simulink model "Modele_LQR_3DOF"  (R2019b)
settings: Solver=VariableStepAuto  StartTime=0.0  StopTime=20  FixedStep=0.1  RelTol=1e-3
undefined symbols (not defined in the file): Amatrix, B, Bmatrix, Fx1, Fx2, Fx3, Fx4, Fx5, Fx6, Fx7, Fx8, Fy1, Fy2, Fy3, Fy4, Fy5, Fy6, Fy7, Fy8, Fz1, Fz2, Fz3, Fz4, Fz5, Fz6, Fz7, Fz8, I_x, I_y, I_z, lx1, lx2, lx3, lx4, lx5, lx6, lx7, lx8, ly1, ly2, ly3, ly4, ly5, ly6, ly7, ly8, lz1, lz2, lz3, lz4, lz5, lz6, lz7, lz8, m, Q, R, W, X0, x_rb ... (+5)
libraries: simulink x12, robotlib x7, dspinverses x1
(part 2 of 2)

== matlab function Modele_LQR_3DOF/ROV model/ROV model/Kinetics1 ==
  data: u input size=1; u_dot output; v input size=1; w input size=1; p input size=1; q input size=1; r input size=1; phi input; theta input; psi input; tau input; v_dot output; w_dot output; p_dot output; q_dot output; r_dot output; u_dot_temp input; v_dot_temp input; w_dot_temp input; p_dot_temp input; q_dot_temp input; r_dot_temp input; disturbance input; EstimatedParams input; B parameter; Fx1 input; Fx2 input; Fx3 input; Fx4 input; Fx5 input; Fx6 input; Fx7 input; Fx8 input; Fy1 input; Fy2 input; Fy3 input; Fy4 input; Fy5 input; Fy6 input; Fy7 input; Fy8 input; Fz1 input; Fz2 input; Fz3 input; Fz4 input; Fz5 input; Fz6 input; Fz7 input; Fz8 input; I_x input; I_y input; I_z input; lx1 input; lx2 input; lx3 input; lx4 input; lx5 input; lx6 input; lx7 input; lx8 input; ly1 input; ly2 input; ly3 input; ly4 input; ly5 input; ly6 input; ly7 input; ly8 input; lz1 input; lz2 input; lz3 input; lz4 input; lz5 input; lz6 input; lz7 input; lz8 input; m parameter; W parameter; x_rb parameter; x_rg parameter; y_rb parameter; y_rg parameter; z_rb parameter; z_rg parameter
function [u_dot,v_dot,w_dot,p_dot,q_dot,r_dot] = Kinetics1(u,v,w,p,q,r,phi,theta,psi,tau,u_dot_temp,v_dot_temp,w_dot_temp,p_dot_temp,q_dot_temp,r_dot_temp, disturbance,EstimatedParams, B, Fx1, Fx2, Fx3, Fx4, Fx5, Fx6, Fx7, Fx8, Fy1, Fy2, Fy3, Fy4, Fy5, Fy6, Fy7, Fy8, Fz1, Fz2, Fz3, Fz4, Fz5, Fz6, Fz7, Fz8, I_x, I_y, I_z, lx1, lx2, lx3, lx4, lx5, lx6, lx7, lx8, ly1, ly2, ly3, ly4, ly5, ly6, ly7, ly8, lz1, lz2, lz3, lz4, lz5, lz6, lz7, lz8, m, W, x_rb, x_rg, y_rb, y_rg, z_rb, z_rg)
% LIVRE HMCH PAGE 58
%extract forces from thrusters
f1=tau(1);
f2=tau(2);
f3=tau(3);
f4=tau(4);
f5=tau(5);
f6=tau(6);
f7=tau(7);
f8=tau(8);

% displaced_water_volume = 0.03;
% water_density = 1000.0;
% m = 24;
% W = -9.81*m;
% B = -W;
%extract estimated parameters
X_u = EstimatedParams(1);
Y_v = EstimatedParams(2);
Z_w = EstimatedParams(3);
K_p = EstimatedParams(4); 
M_q = EstimatedParams(5);
N_r = EstimatedParams(6);
X_uu = EstimatedParams(7);
Y_vv = EstimatedParams(8);
Z_ww = EstimatedParams(9);
K_pp = EstimatedParams(10); 
M_qq = EstimatedParams(11); 
N_rr = EstimatedParams(12);
X_u_dot = EstimatedParams(13);
Y_v_dot = EstimatedParams(14);
Z_w_dot = EstimatedParams(15);
K_p_dot = EstimatedParams(16);
M_q_dot = EstimatedParams(17); 
N_r_dot = EstimatedParams(18); 
%extract forces from disturbance
u_c = disturbance(1);
v_c = disturbance(2);
w_c = disturbance(3);
p_c = disturbance(4);
q_c = disturbance(5);
r_c = disturbance(6);
%Full Equations without disturbance with zg = 0.02
% u_dot = -((0.7071*f1) + (0.7071*f2) - (0.7071*f3) - (0.7071*f4)- (0.230*q_dot_temp) + 2*sin(theta) + u*(X_u + X_uu*abs(u)) - (0.230*p*r) - (11.50*q*w) + (11.50*r*v) - Y_v_dot*r*v + Z_w_dot*q*w)/(X_u_dot - 11.50);
% v_dot = ((0.7071*f1) - (0.7071*f2) + (0.7071*f3) - (0.7071*f4) - (0.230*p_dot_temp) + 2*cos(theta)*sin(phi) - v*(Y_v + Y_vv*abs(v)) + (11.50*q*r) - (11.50*p*w) + (11.50*r*u) - X_u_dot*r*u + Z_w_dot*p*w)/(Y_v_dot - 11.50);
% w_dot = -(f6 - f5 + f7 - f8 - 2*cos(phi)*cos(theta) + w*(Z_w + Z_ww*abs(w)) + q*((23*q)/100 - X_u_dot*u) + p*((23*p)/100 + Y_v_dot*v) - (11.50*p*v) + (11.50*q*u))/(Z_w_dot - 11.50);
% p_dot = -(25*((0.0601*f1) - (0.0601*f2) + (0.0601*f3) - (0.0601*f4) - (109*f5)/500 - (109*f6)/500 + (0.2180*f7) + (0.2180*f8) + (0.230*v_dot_temp) + K_p*p - (2.2560*cos(theta)*sin(phi)) - (0.230*p*w) + (0.230*r*u) - M_q_dot*q*r + N_r_dot*q*r - Y_v_dot*v*w + Z_w_dot*v*w + K_pp*p*abs(p)))/(25*K_p_dot - 4);
% q_dot =-(25*((0.0601*f1) + (0.0601*f2) - (0.0601*f3) - (0.0601*f4)+ (0.120*f5) - (0.120*f6) + (0.120*f7) - (0.120*f8) - (0.230*u_dot_temp) - (2.2560*sin(theta)) + M_q*q - (0.230*q*w) + (0.230*r*v) + K_p_dot*p*r - N_r_dot*p*r + X_u_dot*u*w - Z_w_dot*u*w + M_qq*q*abs(q)))/(25*M_q_dot - 4);
% r_dot = -(25*((0.1888*f2) - (0.1888*f1) + (0.1888*f3) - (0.1888*f4) + N_r*r - K_p_dot*p*q + M_q_dot*p*q - X_u_dot*u*v + Y_v_dot*u*v + N_rr*r*abs(r)))/(25*N_r_dot - 4);

%Full Equations without disturbance with zg = 0.02 + utilisation de la fontion vpa
% u_dot = -(1.0*(0.7071*f1 + 0.7071*f2 - 0.7071*f3 - 0.7071*f4 - 0.23*q_dot_temp + 2.0*sin(theta) + (X_u + X_uu*abs(u - 1.0*u_c))*(u - 1.0*u_c) - 1.0*(11.5*q - 11.5*q_c)*(w - 1.0*w_c) + (11.5*r - 11.5*r_c)*(v - 1.0*v_c) - 1.0*(p - 1.0*p_c)*(0.23*r - 0.23*r_c) + (X_u_dot - 11.5)*(q*w_c - 1.0*r*v_c) - 1.0*Y_v_dot*(r - 1.0*r_c)*(v - 1.0*v_c) + Z_w_dot*(q - 1.0*q_c)*(w - 1.0*w_c)))/(X_u_dot - 11.5);
% v_dot = (0.7071*f1 - 0.7071*f2 + 0.7071*f3 - 0.7071*f4 - 0.23*p_dot_temp - 1.0*(11.5*p - 11.5*p_c)*(w - 1.0*w_c) + (11.5*r - 11.5*r_c)*(u - 1.0*u_c) - 1.0*(Y_v + Y_vv*abs(v - 1.0*v_c))*(v - 1.0*v_c) + 2.0*cos(theta)*sin(phi) + (q - 1.0*q_c)*(0.23*r - 0.23*r_c) + (Y_v_dot - 11.5)*(p*w_c - 1.0*r*u_c) - 1.0*X_u_dot*(r - 1.0*r_c)*(u - 1.0*u_c) + Z_w_dot*(p - 1.0*p_c)*(w - 1.0*w_c))/(Y_v_dot - 11.5);
% w_dot =-(1.0*(f6 - 1.0*f5 + f7 - 1.0*f8 - 1.0*(11.5*p - 11.5*p_c)*(v - 1.0*v_c) + (11.5*q - 11.5*q_c)*(u - 1.0*u_c) - 2.0*cos(phi)*cos(theta) + (Z_w + Z_ww*abs(w - 1.0*w_c))*(w - 1.0*w_c) + (Z_w_dot - 11.5)*(p*v_c - 1.0*q*u_c) + (p - 1.0*p_c)*(0.23*p - 0.23*p_c + Y_v_dot*(v - 1.0*v_c)) - 1.0*(q - 1.0*q_c)*(0.23*q_c - 0.23*q + X_u_dot*(u - 1.0*u_c))))/(Z_w_dot - 11.5);
% p_dot =-(1.0*(0.0601035*f1 - 0.0601035*f2 + 0.0601035*f3 - 0.0601035*f4 - 0.218*f5 - 0.218*f6 + 0.218*f7 + 0.218*f8 + 0.23*v_dot - 2.256*cos(theta)*sin(phi) + (u - 1.0*u_c)*(0.23*r - 0.23*r_c) - 0.23*p*w_c + 0.23*r*u_c - 1.0*(r - 1.0*r_c)*(0.16*q_c - 0.16*q + M_q_dot*(q - 1.0*q_c)) + (q - 1.0*q_c)*(0.16*r_c - 0.16*r + N_r_dot*(r - 1.0*r_c)) + (K_p + K_pp*abs(p - 1.0*p_c))*(p - 1.0*p_c) - 1.0*(w - 1.0*w_c)*(0.23*p - 0.23*p_c + Y_v_dot*(v - 1.0*v_c)) + Z_w_dot*(v - 1.0*v_c)*(w - 1.0*w_c)))/(K_p_dot - 0.16);
% q_dot =-(1.0*(0.0601035*f1 + 0.0601035*f2 - 0.0601035*f3 - 0.0601035*f4 + 0.12*f5 - 0.12*f6 + 0.12*f7 - 0.12*f8 - 0.23*u_dot - 2.256*sin(theta) + (v - 1.0*v_c)*(0.23*r - 0.23*r_c) - 0.23*q*w_c + 0.23*r*v_c + (r - 1.0*r_c)*(0.16*p_c - 0.16*p + K_p_dot*(p - 1.0*p_c)) - 1.0*(p - 1.0*p_c)*(0.16*r_c - 0.16*r + N_r_dot*(r - 1.0*r_c)) + (w - 1.0*w_c)*(0.23*q_c - 0.23*q + X_u_dot*(u - 1.0*u_c)) + (M_q + M_qq*abs(q - 1.0*q_c))*(q - 1.0*q_c) - 1.0*Z_w_dot*(u - 1.0*u_c)*(w - 1.0*w_c)))/(M_q_dot - 0.16);
% r_dot = -(1.0*(0.1887957*f2 - 0.1887957*f1 + 0.1887957*f3 - 0.1887957*f4 - 1.0*(q - 1.0*q_c)*(0.16*p_c - 0.16*p + K_p_dot*(p - 1.0*p_c)) + (p - 1.0*p_c)*(0.16*q_c - 0.16*q + M_q_dot*(q - 1.0*q_c)) + (N_r + N_rr*abs(r - 1.0*r_c))*(r - 1.0*r_c) - 1.0*X_u_dot*(u - 1.0*u_c)*(v - 1.0*v_c) + Y_v_dot*(u - 1.0*u_c)*(v - 1.0*v_c)))/(N_r_dot - 0.16);

% u_dot = -(1.0*((X_u + X_uu*abs(u - 1.0*u_c))*(u - 1.0*u_c) + sin(theta)*(B - 9.81*m) + Fx1*f1 + Fx2*f2 + Fx3*f3 + Fx4*f4 + Fx5*f5 + Fx6*f6 + Fx7*f7 + Fx8*f8 + (q*w_c - 1.0*r*v_c)*(X_u_dot - 1.0*m) + (Z_w_dot*(w - 1.0*w_c) + m*x_rg*(q - 1.0*q_c))*(q - 1.0*q_c) - 1.0*(Y_v_dot*(v - 1.0*v_c) - 1.0*m*x_rg*(r - 1.0*r_c))*(r - 1.0*r_c) - 1.0*(m*y_rg*(q - 1.0*q_c) + m*z_rg*(r - 1.0*r_c))*(p - 1.0*p_c) - 1.0*m*(q - 1.0*q_c)*(w - 1.0*w_c) + m*(r - 1.0*r_c)*(v - 1.0*v_c) - 1.0*m*q_dot_temp*z_rg + m*r_dot_temp*y_rg))/(X_u_dot - 1.0*m);
%  
%  
% v_dot = -(1.0*((Y_v + Y_vv*abs(v - 1.0*v_c))*(v - 1.0*v_c) + Fy1*f1 + Fy2*f2 + Fy3*f3 + Fy4*f4 + Fy5*f5 + Fy6*f6 + Fy7*f7 + Fy8*f8 - 1.0*(p*w_c - 1.0*r*u_c)*(Y_v_dot - 1.0*m) + (X_u_dot*(u - 1.0*u_c) + m*y_rg*(r - 1.0*r_c))*(r - 1.0*r_c) - 1.0*(Z_w_dot*(w - 1.0*w_c) - 1.0*m*y_rg*(p - 1.0*p_c))*(p - 1.0*p_c) - 1.0*(m*x_rg*(p - 1.0*p_c) + m*z_rg*(r - 1.0*r_c))*(q - 1.0*q_c) + m*(p - 1.0*p_c)*(w - 1.0*w_c) - 1.0*m*(r - 1.0*r_c)*(u - 1.0*u_c) + m*p_dot_temp*z_rg - 1.0*m*r_dot_temp*x_rg - 1.0*cos(theta)*sin(phi)*(B - 9.81*m)))/(Y_v_dot - 1.0*m);
%  
%  
% w_dot = -(1.0*(Fz1*f1 + Fz2*f2 + Fz3*f3 + Fz4*f4 + Fz5*f5 + Fz6*f6 + Fz7*f7 + Fz8*f8 + (Z_w + Z_ww*abs(w - 1.0*w_c))*(w - 1.0*w_c) + (p*v_c - 1.0*q*u_c)*(Z_w_dot - 1.0*m) + (Y_v_dot*(v - 1.0*v_c) + m*z_rg*(p - 1.0*p_c))*(p - 1.0*p_c) - 1.0*(X_u_dot*(u - 1.0*u_c) - 1.0*m*z_rg*(q - 1.0*q_c))*(q - 1.0*q_c) - 1.0*(m*x_rg*(p - 1.0*p_c) + m*y_rg*(q - 1.0*q_c))*(r - 1.0*r_c) - 1.0*m*(p - 1.0*p_c)*(v - 1.0*v_c) + m*(q - 1.0*q_c)*(u - 1.0*u_c) - 1.0*m*p_dot_temp*y_rg + m*q_dot_temp*x_rg - 1.0*cos(phi)*cos(theta)*(B - 9.81*m)))/(Z_w_dot - 1.0*m);
%  
%  
% p_dot = -(1.0*((Y_v_dot*(v - 1.0*v_c) + m*z_rg*(p - 1.0*p_c))*(w - 1.0*w_c) + f1*(Fy1*lz1 - 1.0*Fz1*ly1) + f2*(Fy2*lz2 - 1.0*Fz2*ly2) + f3*(Fy3*lz3 - 1.0*Fz3*ly3) + f4*(Fy4*lz4 - 1.0*Fz4*ly4) + f5*(Fy5*lz5 - 1.0*Fz5*ly5) + f6*(Fy6*lz6 - 1.0*Fz6*ly6) + f7*(Fy7*lz7 - 1.0*Fz7*ly7) + f8*(Fy8*lz8 - 1.0*Fz8*ly8) - 1.0*(Z_w_dot*(w - 1.0*w_c) - 1.0*m*y_rg*(p - 1.0*p_c))*(v - 1.0*v_c) - 1.0*(K_p + K_pp*abs(p - 1.0*p_c))*(p - 1.0*p_c) - 1.0*(m*y_rg*(q - 1.0*q_c) + m*z_rg*(r - 1.0*r_c))*(u - 1.0*u_c) - 1.0*(I_y*(q - 1.0*q_c) - 1.0*M_q_dot*(q - 1.0*q_c))*(r - 1.0*r_c) + (I_z*(r - 1.0*r_c) - 1.0*N_r_dot*(r - 1.0*r_c))*(q - 1.0*q_c) + cos(phi)*cos(theta)*(B*y_rb - 9.81*m*y_rg) - 1.0*cos(theta)*sin(phi)*(B*z_rb - 9.81*m*z_rg) + m*y_rg*(w_dot + p*v_c - 1.0*q*u_c) - 1.0*m*z_rg*(v_dot - 1.0*p*w_c + r*u_c)))/(I_x - 1.0*K_p_dot);
%  
%  
% q_dot = (sin(theta)*(B*z_rb - 9.81*m*z_rg) - 1.0*(Z_w_dot*(w - 1.0*w_c) + m*x_rg*(q - 1.0*q_c))*(u - 1.0*u_c) + f1*(Fx1*lz1 - 1.0*Fz1*lx1) + f2*(Fx2*lz2 - 1.0*Fz2*lx2) + f3*(Fx3*lz3 - 1.0*Fz3*lx3) + f4*(Fx4*lz4 - 1.0*Fz4*lx4) + f5*(Fx5*lz5 - 1.0*Fz5*lx5) + f6*(Fx6*lz6 - 1.0*Fz6*lx6) + f7*(Fx7*lz7 - 1.0*Fz7*lx7) + f8*(Fx8*lz8 - 1.0*Fz8*lx8) + (X_u_dot*(u - 1.0*u_c) - 1.0*m*z_rg*(q - 1.0*q_c))*(w - 1.0*w_c) + (M_q + M_qq*abs(q - 1.0*q_c))*(q - 1.0*q_c) - 1.0*(I_x*(p - 1.0*p_c) - 1.0*K_p_dot*(p - 1.0*p_c))*(r - 1.0*r_c) + (m*x_rg*(p - 1.0*p_c) + m*z_rg*(r - 1.0*r_c))*(v - 1.0*v_c) + (I_z*(r - 1.0*r_c) - 1.0*N_r_dot*(r - 1.0*r_c))*(p - 1.0*p_c) + cos(phi)*cos(theta)*(B*x_rb - 9.81*m*x_rg) + m*x_rg*(w_dot + p*v_c - 1.0*q*u_c) - 1.0*m*z_rg*(u_dot + q*w_c - 1.0*r*v_c))/(I_y - 1.0*M_q_dot);
%  
%  
% r_dot = -(1.0*(sin(theta)*(B*y_rb - 9.81*m*y_rg) + (X_u_dot*(u - 1.0*u_c) + m*y_rg*(r - 1.0*r_c))*(v - 1.0*v_c) + f1*(Fx1*ly1 - 1.0*Fy1*lx1) + f2*(Fx2*ly2 - 1.0*Fy2*lx2) + f3*(Fx3*ly3 - 1.0*Fy3*lx3) + f4*(Fx4*ly4 - 1.0*Fy4*lx4) + f5*(Fx5*ly5 - 1.0*Fy5*lx5) + f6*(Fx6*ly6 - 1.0*Fy6*lx6) + f7*(Fx7*ly7 - 1.0*Fy7*lx7) + f8*(Fx8*ly8 - 1.0*Fy8*lx8) - 1.0*(Y_v_dot*(v - 1.0*v_c) - 1.0*m*x_rg*(r - 1.0*r_c))*(u - 1.0*u_c) - 1.0*(N_r + N_rr*abs(r - 1.0*r_c))*(r - 1.0*r_c) - 1.0*(I_x*(p - 1.0*p_c) - 1.0*K_p_dot*(p - 1.0*p_c))*(q - 1.0*q_c) + (I_y*(q - 1.0*q_c) - 1.0*M_q_dot*(q - 1.0*q_c))*(p - 1.0*p_c) - 1.0*(m*x_rg*(p - 1.0*p_c) + m*y_rg*(q - 1.0*q_c))*(w - 1.0*w_c) + cos(theta)*sin(phi)*(B*x_rb - 9.81*m*x_rg) + m*x_rg*(v_dot - 1.0*p*w_c + r*u_c) - 1.0*m*y_rg*(u_dot + q*w_c - 1.0*r*v_c)))/(I_z - 1.0*N_r_dot);
 
u_dot = -(1.0*((X_u + X_uu*abs(u - 1.0*u_c))*(u - 1.0*u_c) + Fx1*f1 + Fx2*f2 + Fx3*f3 + Fx4*f4 + Fx5*f5 + Fx6*f6 + Fx7*f7 + Fx8*f8 + (q*w_c - 1.0*r*v_c)*(X_u_dot - 1.0*m) + (Z_w_dot*(w - 1.0*w_c) + m*x_rg*(q - 1.0*q_c))*(q - 1.0*q_c) - 1.0*(Y_v_dot*(v - 1.0*v_c) - 1.0*m*x_rg*(r - 1.0*r_c))*(r - 1.0*r_c) + sin(theta)*(B - 1.0*W) - 1.0*(m*y_rg*(q - 1.0*q_c) + m*z_rg*(r - 1.0*r_c))*(p - 1.0*p_c) - 1.0*m*(q - 1.0*q_c)*(w - 1.0*w_c) + m*(r - 1.0*r_c)*(v - 1.0*v_c) - 1.0*m*q_dot_temp*z_rg + m*r_dot_temp*y_rg))/(X_u_dot - 1.0*m);

 
v_dot = -(1.0*((Y_v + Y_vv*abs(v - 1.0*v_c))*(v - 1.0*v_c) + Fy1*f1 + Fy2*f2 + Fy3*f3 + Fy4*f4 + Fy5*f5 + Fy6*f6 + Fy7*f7 + Fy8*f8 - 1.0*(p*w_c - 1.0*r*u_c)*(Y_v_dot - 1.0*m) + (X_u_dot*(u - 1.0*u_c) + m*y_rg*(r - 1.0*r_c))*(r - 1.0*r_c) - 1.0*(Z_w_dot*(w - 1.0*w_c) - 1.0*m*y_rg*(p - 1.0*p_c))*(p - 1.0*p_c) - 1.0*(m*x_rg*(p - 1.0*p_c) + m*z_rg*(r - 1.0*r_c))*(q - 1.0*q_c) + m*(p - 1.0*p_c)*(w - 1.0*w_c) - 1.0*m*(r - 1.0*r_c)*(u - 1.0*u_c) - 1.0*cos(theta)*sin(phi)*(B - 1.0*W) + m*p_dot_temp*z_rg - 1.0*m*r_dot_temp*x_rg))/(Y_v_dot - 1.0*m);


w_dot = -(1.0*(Fz1*f1 + Fz2*f2 + Fz3*f3 + Fz4*f4 + Fz5*f5 + Fz6*f6 + Fz7*f7 + Fz8*f8 + (Z_w + Z_ww*abs(w - 1.0*w_c))*(w - 1.0*w_c) + (p*v_c - 1.0*q*u_c)*(Z_w_dot - 1.0*m) + (Y_v_dot*(v - 1.0*v_c) + m*z_rg*(p - 1.0*p_c))*(p - 1.0*p_c) - 1.0*(X_u_dot*(u - 1.0*u_c) - 1.0*m*z_rg*(q - 1.0*q_c))*(q - 1.0*q_c) - 1.0*(m*x_rg*(p - 1.0*p_c) + m*y_rg*(q - 1.0*q_c))*(r - 1.0*r_c) - 1.0*m*(p - 1.0*p_c)*(v - 1.0*v_c) + m*(q - 1.0*q_c)*(u - 1.0*u_c) - 1.0*cos(phi)*cos(theta)*(B - 1.0*W) - 1.0*m*p_dot_temp*y_rg + m*q_dot_temp*x_rg))/(Z_w_dot - 1.0*m);

 
p_dot = -(1.0*((Y_v_dot*(v - 1.0*v_c) + m*z_rg*(p - 1.0*p_c))*(w - 1.0*w_c) - 1.0*cos(theta)*(W*y_rg*cos(phi) - 1.0*W*z_rg*sin(phi) - 1.0*B*y_rb*cos(phi) + B*z_rb*sin(phi)) + f1*(Fy1*lz1 - 1.0*Fz1*ly1) + f2*(Fy2*lz2 - 1.0*Fz2*ly2) + f3*(Fy3*lz3 - 1.0*Fz3*ly3) + f4*(Fy4*lz4 - 1.0*Fz4*ly4) + f5*(Fy5*lz5 - 1.0*Fz5*ly5) + f6*(Fy6*lz6 - 1.0*Fz6*ly6) + f7*(Fy7*lz7 - 1.0*Fz7*ly7) + f8*(Fy8*lz8 - 1.0*Fz8*ly8) - 1.0*(Z_w_dot*(w - 1.0*w_c) - 1.0*m*y_rg*(p - 1.0*p_c))*(v - 1.0*v_c) - 1.0*(K_p + K_pp*abs(p - 1.0*p_c))*(p - 1.0*p_c) - 1.0*(m*y_rg*(q - 1.0*q_c) + m*z_rg*(r - 1.0*r_c))*(u - 1.0*u_c) - 1.0*(I_y*(q - 1.0*q_c) - 1.0*M_q_dot*(q - 1.0*q_c))*(r - 1.0*r_c) + (I_z*(r - 1.0*r_c) - 1.0*N_r_dot*(r - 1.0*r_c))*(q - 1.0*q_c) + m*y_rg*(w_dot + p*v_c - 1.0*q*u_c) - 1.0*m*z_rg*(v_dot - 1.0*p*w_c + r*u_c)))/(I_x - 1.0*K_p_dot);

 
q_dot = (f1*(Fx1*lz1 - 1.0*Fz1*lx1) - 1.0*(Z_w_dot*(w - 1.0*w_c) + m*x_rg*(q - 1.0*q_c))*(u - 1.0*u_c) + f2*(Fx2*lz2 - 1.0*Fz2*lx2) + f3*(Fx3*lz3 - 1.0*Fz3*lx3) + f4*(Fx4*lz4 - 1.0*Fz4*lx4) + f5*(Fx5*lz5 - 1.0*Fz5*lx5) + f6*(Fx6*lz6 - 1.0*Fz6*lx6) + f7*(Fx7*lz7 - 1.0*Fz7*lx7) + f8*(Fx8*lz8 - 1.0*Fz8*lx8) + (X_u_dot*(u - 1.0*u_c) - 1.0*m*z_rg*(q - 1.0*q_c))*(w - 1.0*w_c) + (M_q + M_qq*abs(q - 1.0*q_c))*(q - 1.0*q_c) - 1.0*(I_x*(p - 1.0*p_c) - 1.0*K_p_dot*(p - 1.0*p_c))*(r - 1.0*r_c) + (m*x_rg*(p - 1.0*p_c) + m*z_rg*(r - 1.0*r_c))*(v - 1.0*v_c) + (I_z*(r - 1.0*r_c) - 1.0*N_r_dot*(r - 1.0*r_c))*(p - 1.0*p_c) + B*z_rb*sin(theta) - 1.0*W*z_rg*sin(theta) + m*x_rg*(w_dot + p*v_c - 1.0*q*u_c) - 1.0*m*z_rg*(u_dot + q*w_c - 1.0*r*v_c) + B*x_rb*cos(phi)*cos(theta) - 1.0*W*x_rg*cos(phi)*cos(theta))/(I_y - 1.0*M_q_dot);
 
 
r_dot = -(1.0*((X_u_dot*(u - 1.0*u_c) + m*y_rg*(r - 1.0*r_c))*(v - 1.0*v_c) + f1*(Fx1*ly1 - 1.0*Fy1*lx1) + f2*(Fx2*ly2 - 1.0*Fy2*lx2) + f3*(Fx3*ly3 - 1.0*Fy3*lx3) + f4*(Fx4*ly4 - 1.0*Fy4*lx4) + f5*(Fx5*ly5 - 1.0*Fy5*lx5) + f6*(Fx6*ly6 - 1.0*Fy6*lx6) + f7*(Fx7*ly7 - 1.0*Fy7*lx7) + f8*(Fx8*ly8 - 1.0*Fy8*lx8) - 1.0*(Y_v_dot*(v - 1.0*v_c) - 1.0*m*x_rg*(r - 1.0*r_c))*(u - 1.0*u_c) - 1.0*(N_r + N_rr*abs(r - 1.0*r_c))*(r - 1.0*r_c) - 1.0*(I_x*(p - 1.0*p_c) - 1.0*K_p_dot*(p - 1.0*p_c))*(q - 1.0*q_c) + (I_y*(q - 1.0*q_c) - 1.0*M_q_dot*(q - 1.0*q_c))*(p - 1.0*p_c) - 1.0*(m*x_rg*(p - 1.0*p_c) + m*y_rg*(q - 1.0*q_c))*(w - 1.0*w_c) + B*y_rb*sin(theta) - 1.0*W*y_rg*sin(theta) + m*x_rg*(v_dot - 1.0*p*w_c + r*u_c) - 1.0*m*y_rg*(u_dot + q*w_c - 1.0*r*v_c) + B*x_rb*cos(theta)*sin(phi) - 1.0*W*x_rg*cos(theta)*sin(phi)))/(I_z - 1.0*N_r_dot);
end

== matlab function Modele_LQR_3DOF/controller/MATLAB Function ==
  data: Q output; R output; state input; A output; B output
function [Q,R,A,B]= ABmatrix(state)

y = u;

== matlab function Modele_LQR_3DOF/Thrustherforces in newtons/toPWM/MATLAB Function ==
  data: blankMessage input Bus: SL_Bus_DOF_6_lin_velocity_v3_ActuatorThrottle_os1e1p; msg output; data input
function msg = assignArray(blankMessage,data)
blankMessage.Ids = uint8([0 1 2 3 4 5 6 7]');
blankMessage.Ids_SL_Info.CurrentLength = uint32(8);
blankMessage.Ids_SL_Info.ReceivedLength = uint32(8);
blankMessage.Throttles = data;
blankMessage.Throttles_SL_Info.CurrentLength = uint32(8);
blankMessage.Throttles_SL_Info.ReceivedLength = uint32(8);
msg = blankMessage;
end

== matlab function Modele_LQR_3DOF/ROV model/ROV model/Kinematics ==
  data: u_b input; u_n output; v_b input; w_b input; p_b input; q_b input; r_b input; phi input; theta input; psi input; v_n output; w_n output; p_n output; q_n output; r_n output
function [u_n,v_n,w_n,p_n,q_n,r_n] = Kinematics(u_b,v_b,w_b,p_b,q_b,r_b,phi,theta,psi)
% LIVRE HMCH PAGE 27
cphi = cos(phi);
sphi = sin(phi);
cth  = cos(theta);
sth  = sin(theta);
cpsi = cos(psi);
spsi = sin(psi);
tanth = tan(theta);
if cth==0
    error('T is singular for theta = +-90 degrees');
end
 
u_n = u_b*cpsi*cth + v_b*(cpsi*sphi*sth - cphi*spsi) + w_b*(sphi*spsi + cphi*cpsi*sth) ;
v_n = u_b*cth*spsi + v_b*(cphi*cpsi + sphi*spsi*sth) + w_b*(cphi*spsi*sth - cpsi*sphi);
w_n = -u_b*sth+ v_b*cth*sphi + w_b*cphi*cth;
p_n = p_b + q_b*sphi*(tanth) + r_b*cphi*(tanth);
q_n = q_b*cphi - r_b*sphi;
r_n = q_b*(sphi/cth) + r_b*(cphi/cth);

% u_n =  w_b*(sphi*spsi + cphi*cpsi*sth) - v_b*(cphi*spsi - cpsi*sphi*sth) + u_b*cpsi*cth;
% v_n =  v_b*(cphi*cpsi + sphi*spsi*sth) - w_b*(cpsi*sphi - cphi*spsi*sth) + u_b*cth*spsi;
% w_n = w_b*cphi*cth - u_b*sth + v_b*cth*sphi;
% p_n = p_b + (r_b*cphi*sth)/cth + (q_b*sphi*sth)/cth;
% q_n = q_b*cphi - r_b*sphi;
% r_n = (r_b*cphi)/cth + (q_b*sphi)/cth;
end

== matlab function Modele_LQR_3DOF/controller/LQR/MATLAB Function ==
  data: dXdt output; X input; A input; B input; R input; Q input
function dXdt  = mRiccati(X, A, B,R,Q)
% r1=randi([1 1000]);
% r2=randi([1 1000]);
% r3=randi([1 1000]);
% r4=randi([1 1000]);
% r5=randi([1 1000]);
% r6=randi([1 1000]);
% Q = diag([r1 r2 r3 r4 r5 r6] );
% R = 1*diag([1 1 1 1]);
%X = reshape(X, size(A)); %Convert from "n^2"-by-1 to "n"-by-"n"
dXdt = A.'*X + X*A - (X*B)*inv(R)*(B.'*X) + Q; %Determine derivative
% dXdtS= dXdt(:); %Convert from "n"-by-"n" to "n^2"-by-1,algebraic Riccati equation (ARE)

== matlab function Modele_LQR_3DOF/Subsystem/Simulation/p_sin2/sin_fcn ==
  data: amplitude input; y output; frequency input; bias input; time input; start_time input; end_time input
function y = fcn(amplitude, frequency, bias, time, start_time, end_time)
%#codegen
if ( time < start_time)
    y = bias;
elseif ( start_time <= time & time <= end_time + start_time) 
    y = amplitude*sin(2*pi*frequency*(time-start_time)) + bias;
else
    y = amplitude*sin(2*pi*frequency*(end_time+start_time)) + bias;
end

end

== matlab function Modele_LQR_3DOF/Subsystem/Simulation/p_step1/step_fcn ==
  data: q0 input; traj output; qf input; t input; ts input; tf input; V_scaling input
function traj   = smoothStep(q0, qf, t, ts, tf, V_scaling)
%#codegen
V = V_scaling*(qf - q0)/(tf - ts);

tb = (q0 - qf + V*(tf - ts))/V;
alfa = V/tb;
if ( t < ts)
    traj = q0;
elseif (0 <= (t - ts) & (t - ts) <= tb)
    traj = q0 + alfa*(t - ts)^2/2;
elseif (tb < (t - ts) & (t - ts) <= (tf - ts) - tb)
    traj = (qf + q0 - V*(tf - ts))/2 + V*(t - ts);
elseif (tf - ts - tb < (t - ts) & (t - ts) <= (tf - ts))
    traj = qf - alfa*(tf - ts)^2/2 + alfa*(tf - ts)*(t - ts) - alfa*(t - ts)^2/2;
else
    traj = qf;
end

end

== matlab function Modele_LQR_3DOF/Subsystem/Simulation/p_step2/step_fcn ==
  data: q0 input; traj output; qf input; t input; ts input; tf input; V_scaling input
function traj   = smoothStep(q0, qf, t, ts, tf, V_scaling)
%#codegen
V = V_scaling*(qf - q0)/(tf - ts);

tb = (q0 - qf + V*(tf - ts))/V;
alfa = V/tb;
if ( t < ts)
    traj = q0;
elseif (0 <= (t - ts) & (t - ts) <= tb)
    traj = q0 + alfa*(t - ts)^2/2;
elseif (tb < (t - ts) & (t - ts) <= (tf - ts) - tb)
    traj = (qf + q0 - V*(tf - ts))/2 + V*(t - ts);
elseif (tf - ts - tb < (t - ts) & (t - ts) <= (tf - ts))
    traj = qf - alfa*(tf - ts)^2/2 + alfa*(tf - ts)*(t - ts) - alfa*(t - ts)^2/2;
else
    traj = qf;
end

end

== matlab function Modele_LQR_3DOF/Subsystem/Simulation/p_step3/step_fcn ==
  data: q0 input; traj output; qf input; t input; ts input; tf input; V_scaling input
function traj   = smoothStep(q0, qf, t, ts, tf, V_scaling)
%#codegen
V = V_scaling*(qf - q0)/(tf - ts);

tb = (q0 - qf + V*(tf - ts))/V;
alfa = V/tb;
if ( t < ts)
    traj = q0;
elseif (0 <= (t - ts) & (t - ts) <= tb)
    traj = q0 + alfa*(t - ts)^2/2;
elseif (tb < (t - ts) & (t - ts) <= (tf - ts) - tb)
    traj = (qf + q0 - V*(tf - ts))/2 + V*(t - ts);
elseif (tf - ts - tb < (t - ts) & (t - ts) <= (tf - ts))
    traj = qf - alfa*(tf - ts)^2/2 + alfa*(tf - ts)*(t - ts) - alfa*(t - ts)^2/2;
else
    traj = qf;
end

end

== matlab function Modele_LQR_3DOF/Subsystem/Simulation/p_sin4/sin_fcn ==
  data: amplitude input; y output; frequency input; bias input; time input; start_time input; end_time input
function y = fcn(amplitude, frequency, bias, time, start_time, end_time)
%#codegen
if ( time < start_time)
    y = bias;
elseif ( start_time <= time & time <= end_time + start_time) 
    y = amplitude*sin(2*pi*frequency*(time-start_time)) + bias;
else
    y = amplitude*sin(2*pi*frequency*(end_time+start_time)) + bias;
end

end

== matlab function Modele_LQR_3DOF/Subsystem/Simulation/p_step4/step_fcn ==
  data: q0 input; traj output; qf input; t input; ts input; tf input; V_scaling input
function traj   = smoothStep(q0, qf, t, ts, tf, V_scaling)
%#codegen
V = V_scaling*(qf - q0)/(tf - ts);

tb = (q0 - qf + V*(tf - ts))/V;
alfa = V/tb;
if ( t < ts)
    traj = q0;
elseif (0 <= (t - ts) & (t - ts) <= tb)
    traj = q0 + alfa*(t - ts)^2/2;
elseif (tb < (t - ts) & (t - ts) <= (tf - ts) - tb)
    traj = (qf + q0 - V*(tf - ts))/2 + V*(t - ts);
elseif (tf - ts - tb < (t - ts) & (t - ts) <= (tf - ts))
    traj = qf - alfa*(tf - ts)^2/2 + alfa*(tf - ts)*(t - ts) - alfa*(t - ts)^2/2;
else
    traj = qf;
end

end

== matlab function Modele_LQR_3DOF/Subsystem/Simulation/p_sin5/sin_fcn ==
  data: amplitude input; y output; frequency input; bias input; time input; start_time input; end_time input
function y = fcn(amplitude, frequency, bias, time, start_time, end_time)
%#codegen
if ( time < start_time)
    y = bias;
elseif ( start_time <= time & time <= end_time + start_time) 
    y = amplitude*sin(2*pi*frequency*(time-start_time)) + bias;
else
    y = amplitude*sin(2*pi*frequency*(end_time+start_time)) + bias;
end

end

== matlab function Modele_LQR_3DOF/Subsystem/Simulation/p_step5/step_fcn ==
  data: q0 input; traj output; qf input; t input; ts input; tf input; V_scaling input
function traj   = smoothStep(q0, qf, t, ts, tf, V_scaling)
%#codegen
V = V_scaling*(qf - q0)/(tf - ts);

tb = (q0 - qf + V*(tf - ts))/V;
alfa = V/tb;
if ( t < ts)
    traj = q0;
elseif (0 <= (t - ts) & (t - ts) <= tb)
    traj = q0 + alfa*(t - ts)^2/2;
elseif (tb < (t - ts) & (t - ts) <= (tf - ts) - tb)
    traj = (qf + q0 - V*(tf - ts))/2 + V*(t - ts);
elseif (tf - ts - tb < (t - ts) & (t - ts) <= (tf - ts))
    traj = qf - alfa*(tf - ts)^2/2 + alfa*(tf - ts)*(t - ts) - alfa*(t - ts)^2/2;
else
    traj = qf;
end

end

== matlab function Modele_LQR_3DOF/Subsystem/Simulation/p_sin6/sin_fcn ==
  data: amplitude input; y output; frequency input; bias input; time input; start_time input; end_time input
function y = fcn(amplitude, frequency, bias, time, start_time, end_time)
%#codegen
if ( time < start_time)
    y = bias;
elseif ( start_time <= time & time <= end_time + start_time) 
    y = amplitude*sin(2*pi*frequency*(time-start_time)) + bias;
else
    y = amplitude*sin(2*pi*frequency*(end_time+start_time)) + bias;
end

end

== matlab function Modele_LQR_3DOF/Subsystem/Simulation/p_step6/step_fcn ==
  data: q0 input; traj output; qf input; t input; ts input; tf input; V_scaling input
function traj   = smoothStep(q0, qf, t, ts, tf, V_scaling)
%#codegen
V = V_scaling*(qf - q0)/(tf - ts);

tb = (q0 - qf + V*(tf - ts))/V;
alfa = V/tb;
if ( t < ts)
    traj = q0;
elseif (0 <= (t - ts) & (t - ts) <= tb)
    traj = q0 + alfa*(t - ts)^2/2;
elseif (tb < (t - ts) & (t - ts) <= (tf - ts) - tb)
    traj = (qf + q0 - V*(tf - ts))/2 + V*(t - ts);
elseif (tf - ts - tb < (t - ts) & (t - ts) <= (tf - ts))
    traj = qf - alfa*(tf - ts)^2/2 + alfa*(tf - ts)*(t - ts) - alfa*(t - ts)^2/2;
else
    traj = qf;
end

end

== matlab function Modele_LQR_3DOF/Subsystem/Simulation/p_sin7/sin_fcn ==
  data: amplitude input; y output; frequency input; bias input; time input; start_time input; end_time input
function y = fcn(amplitude, frequency, bias, time, start_time, end_time)
%#codegen
if ( time < start_time)
    y = bias;
elseif ( start_time <= time & time <= end_time + start_time) 
    y = amplitude*sin(2*pi*frequency*(time-start_time)) + bias;
else
    y = amplitude*sin(2*pi*frequency*(end_time+start_time)) + bias;
end

end

== matlab function Modele_LQR_3DOF/Thrustherforces in newtons/MATLAB Function1 ==
  data: u input; k output
function k  = Normalize(u)
k = (u-1500)*150/400;
end

== matlab function Modele_LQR_3DOF/controller/MATLAB Function1 ==
  data: x input; y input; z input; u input; v output
function v = add_vitesse(x,y,z,u)
    v = [0;0;0;0;0;0;0;0];
    vitesse = [x;y;z;0;0;0];
    thrust_position = [    0.2987,  0.2130, 0;  %thruster 1
                           0.2987, -0.2130, 0;  %thruster 2
                          -0.1073,  0.2725, 0;  %thruster 3
                          -0.1073, -0.2725, 0;  %thruster 4
                           0.1073,  0.2725, 0;  %thruster 5
                           0.1073, -0.2725, 0;  %thruster 6
                          -0.2987,  0.2130, 0;  %thruster 7
                          -0.2987, -0.2130, 0]; %thruster 8
     
    thrust_direction = [     0.707,   -0.707,    0;   %thruster 1
                             0.707,    0.707,    0;   %thruster 2
                             0.0,      0.0,      1;   %thruster 3
                             0.0,      0.0,     -1;   %thruster 4
                             0.0,      0.0,      1;   %thruster 5
                             0.0,      0.0,      1;   %thruster 6
                             0.707,    0.707,    0;   %thruster 7
                             0.707,   -0.707,    0];  %thruster 8
      thrust_allocation = zeros(8,6);
      thrust_allocation(1:8,1:3) = thrust_direction; %map XYZ Froces
      
      for i = 1:8
           thrust_allocation(i,4:6) = cross(thrust_position(i,1:3),thrust_direction(i,1:3)); %maps XYZ torques
      end
      lin = [0;0;0;0;0;0;0;0];
      lin = thrust_allocation*vitesse;
      v = lin + u;
      
end

== matlab function Modele_LQR_3DOF/Subsystem/Simulation/p_step7/step_fcn ==
  data: q0 input; traj output; qf input; t input; ts input; tf input; V_scaling input
function traj   = smoothStep(q0, qf, t, ts, tf, V_scaling)
%#codegen
V = V_scaling*(qf - q0)/(tf - ts);

tb = (q0 - qf + V*(tf - ts))/V;
alfa = V/tb;
if ( t < ts)
    traj = q0;
elseif (0 <= (t - ts) & (t - ts) <= tb)
    traj = q0 + alfa*(t - ts)^2/2;
elseif (tb < (t - ts) & (t - ts) <= (tf - ts) - tb)
    traj = (qf + q0 - V*(tf - ts))/2 + V*(t - ts);
elseif (tf - ts - tb < (t - ts) & (t - ts) <= (tf - ts))
    traj = qf - alfa*(tf - ts)^2/2 + alfa*(tf - ts)*(t - ts) - alfa*(t - ts)^2/2;
else
    traj = qf;
end

end

== matlab function Modele_LQR_3DOF/Thrustherforces in newtons/MATLAB Function2 ==
  data: u input; tau output
function tau = fcn(u)
%#codegen
lookup =[...
    -40.0337   -1.0000
    -40.0337   -0.9750
    -40.0788   -0.9500
    -37.5428   -0.9250
    -36.6092   -0.9000
    -35.4971   -0.8750
    -33.7623   -0.8500
    -32.3835   -0.8250
    -31.2263   -0.8000
    -29.9809   -0.7750
    -28.5128   -0.7500
    -27.6234   -0.7250
    -26.5554   -0.7000
    -24.7765   -0.6750
    -23.1751   -0.6500
    -22.1522   -0.6250
    -21.3510   -0.6000
    -19.5280   -0.5750
    -18.4600   -0.5500
    -17.3480   -0.5250
    -16.1025   -0.5000
    -14.6345   -0.4750
    -13.0781   -0.4500
    -12.1877   -0.4250
    -10.9874   -0.4000
    -10.0528   -0.3750
    -8.8966   -0.3500
    -7.7404   -0.3250
    -6.8058   -0.3000
    -6.0497   -0.2750
    -5.1151   -0.2500
    -4.2698   -0.2250
    -3.4696   -0.2000
    -2.7135   -0.1750
    -1.8682   -0.1500
    -1.1121   -0.1250
    -0.5335   -0.1000
    -0.2667   -0.0750
    0   -0.0500
    0   -0.0250
    0         0
    0    0.0250
    0    0.0500
    0.5786    0.0750
    1.1121    0.1000
    1.8240    0.1250
    2.5801    0.1500
    3.4255    0.1750
    4.0923    0.2000
    5.1151    0.2250
    6.2272    0.2500
    7.0284    0.2750
    8.2739    0.3000
    9.2526    0.3250
    10.8089    0.3500
    12.2328    0.3750
    13.6558    0.4000
    14.9904    0.4250
    16.4585    0.4500
    17.7039    0.4750
    19.2161    0.5000
    20.5508    0.5250
    21.7521    0.5500
    23.6644    0.5750
    24.7324    0.6000
    26.4221    0.6250
    27.7126    0.6500
    29.6249    0.6750
    31.3156    0.7000
    32.8729    0.7250
    33.8065    0.7500
    34.2517    0.7750
    37.0534    0.8000
    38.6549    0.8250
    39.2776    0.8500
    41.1458    0.8750
    42.9257    0.9000
    44.7938    0.9250
    47.1062    0.9500
    48.0408    0.9750
    49.9531    1.0000];
%Thrustherforce in newtons.
tau = zeros(8,1);
tau(1) = interp1(lookup(:,2),lookup(:,1),u(1));
tau(2) = interp1(lookup(:,2),lookup(:,1),u(2));
tau(3) = interp1(lookup(:,2),lookup(:,1),u(3));
tau(4) = interp1(lookup(:,2),lookup(:,1),u(4));
tau(5) = interp1(lookup(:,2),lookup(:,1),u(5));
tau(6) = interp1(lookup(:,2),lookup(:,1),u(6));
tau(7) = interp1(lookup(:,2),lookup(:,1),u(7));
tau(8) = interp1(lookup(:,2),lookup(:,1),u(8));

end
